simulink model "RobotArmSimulator"  (Simulink 7.7)
settings: Solver=ode45  StartTime=0.0  StopTime=10.0  RelTol=1e-3
libraries: vrlib x1
settings Model: Creator=Owner  LastModifiedBy=Owner

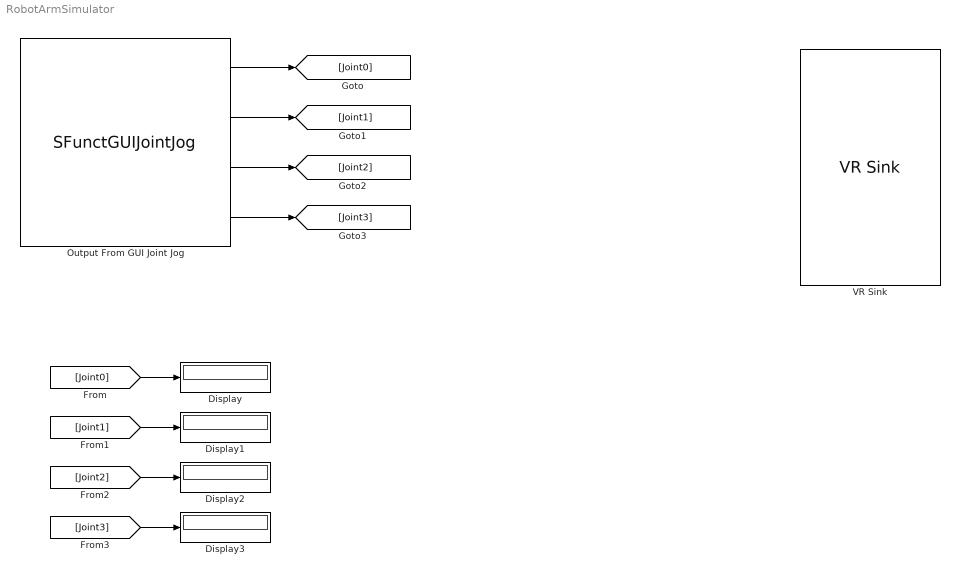
== system RobotArmSimulator ==
  Display{,1..3} (4 alike) : Display
  Output From GUI Joint Jog : M-S-Function  FunctionName=SFunctGUIJointJog
      mask Display:
      | port_label('output', 1, 'Joint Jog 0')
      | port_label('output', 2, 'Joint Jog 1')
      | port_label('output', 3, 'Joint Jog 2')
      | port_label('output', 4, 'Joint Jog 3')
      | disp('GUI Join Jog')
  VR Sink : vrlib/VR Sink  SampleTime=0.01  ViewEnable=on  RemoteChange=off  RemoteView=on  FieldsWritten=RoboticArm.rotation.4.1.1.double  WorldFileName=arm3d2.wrl  AutoView=off  VideoDimensions=[]
  wires:
  Output From GUI Joint Jog/1 -> [Joint0]
  [Joint0] -> Display/1
  Output From GUI Joint Jog/2 -> [Joint1]
  Output From GUI Joint Jog/3 -> [Joint2]
  Output From GUI Joint Jog/4 -> [Joint3]
  [Joint1] -> Display1/1
  [Joint2] -> Display2/1
  [Joint3] -> Display3/1
